simulink library "inp"  (R2021b)
settings: Solver=VariableStepAuto  StartTime=0.0  StopTime=10.0  RelTol=1e-3
undefined symbols (not defined in the file): C_TASK_5MS_S, FALSE, KINP_AcoreReadyToSlp_flg_ovrdflg, KINP_AcoreReadyToSlp_flg_ovrdval, KINP_AllowMovThd_OTA_enum_ovrdflg, KINP_AllowMovThd_OTA_enum_ovrdval, KINP_APSAngleTarget_Deg_ovrdflg, KINP_APSAngleTarget_Deg_ovrdval, KINP_APSDecReq_mps2_ovrdflg, KINP_APSDecReq_mps2_ovrdval, KINP_APSDecReqA_flg_ovrdflg, KINP_APSDecReqA_flg_ovrdval, KINP_APSDFLL_cm_ovrdflg, KINP_APSDFLL_cm_ovrdval, KINP_APSDFLR_cm_ovrdflg, KINP_APSDFLR_cm_ovrdval, KINP_APSDRLL_cm_ovrdflg, KINP_APSDRLL_cm_ovrdval, KINP_APSDRLR_cm_ovrdflg, KINP_APSDRLR_cm_ovrdval, KINP_APSExitCondition_enum_ovrdflg, KINP_APSExitCondition_enum_ovrdval, KINP_APSHWVer_enum_ovrdflg, KINP_APSHWVer_enum_ovrdval, KINP_APSProgressPCT_pct_ovrdflg, KINP_APSProgressPCT_pct_ovrdval, KINP_APSPwrReq_enum_ovrdflg, KINP_APSPwrReq_enum_ovrdval, KINP_APSReq_enum_ovrdflg, KINP_APSReq_enum_ovrdval, KINP_APSRQDisplay_enum_ovrdflg, KINP_APSRQDisplay_enum_ovrdval, KINP_APSRqEPASCtrl_flg_ovrdflg, KINP_APSRqEPASCtrl_flg_ovrdval, KINP_APSShiftPosnReq_enum_ovrdval, KINP_APSShiftPosnReq_enum_ovrflg, KINP_APSSpeedCMD_kph_ovrdval, KINP_APSSpeedCMD_kph_ovrflg, KINP_APSStaSystem_enum_ovrdflg, KINP_APSStaSystem_enum_ovrdval, KINP_APSSWVer_enum_ovrdflg, KINP_APSSWVer_enum_ovrdval, KINP_APSVMCReqA_flg_ovrdval, KINP_APSVMCReqA_flg_ovrflg, KINP_APSVRqEPASCtrl_flg_ovrdflg, KINP_APSVRqEPASCtrl_flg_ovrdval, KINP_AuxBattVolmV_mV_ovrdflg, KINP_AuxBattVolmV_mV_ovrdval, KINP_BTConnectSta_enum_ovrdflg, KINP_BTConnectSta_enum_ovrdval, KINP_CAASSta_enum_ovrdflg, KINP_CAASSta_enum_ovrdval, KINP_CAASVMCReqA_flg_ovrdval, KINP_CAASVMCReqA_flg_ovrflg, KINP_CAN1BusOff_flg_ovrdflg, KINP_CAN1BusOff_flg_ovrdval, KINP_CAN2BusOff_flg_ovrdflg, KINP_CAN2BusOff_flg_ovrdval, KINP_CAN3BusOff_flg_ovrdflg, KINP_CAN3BusOff_flg_ovrdval ... (+158)
libraries: FVT_lib x184, hcu_lib x1
(part 5 of 8)

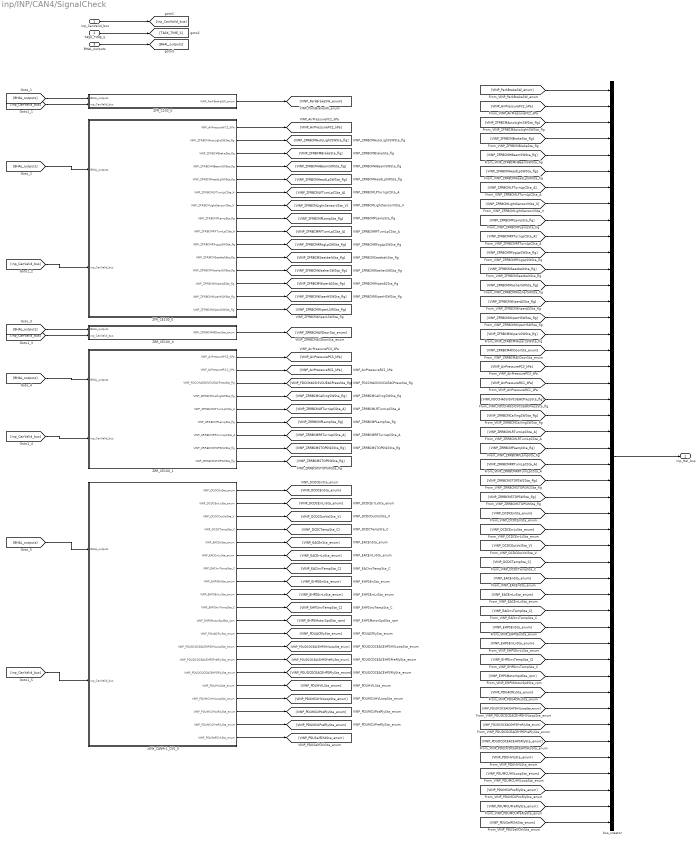
== system inp/INP/CAN4/SignalCheck ==
  inp_CanValid_bus : Inport
  TASK_TIME_S : Inport  Port=2
  BHAL_outputs : Inport  Port=3
  ZFR_C100_0 : Subsystem
  ZFR_CE100_0 : Subsystem
  ZRR_CE100_0 : Subsystem
  ZRR_CE100_1 : Subsystem
  bus_creator : BusCreator  Inputs=46
  zGW_CANRr1_C50_0 : Subsystem
  inp_Hal_bus : Outport
  wires:
  inp_CanValid_bus/1 -> [inp_CanValid_bus]
  TASK_TIME_S/1 -> [TASK_TIME_S]
  BHAL_outputs/1 -> [BHAL_outputs]
  [BHAL_outputs] -> ZFR_C100_0/1(BHAL_outputs)
  [inp_CanValid_bus] -> ZFR_C100_0/2(inp_CanValid_bus)
  ZFR_C100_0/1(VINP_ParkBrakeSW_enum) -> [VINP_ParkBrakeSW_enum]
  [BHAL_outputs] -> ZFR_CE100_0/1(BHAL_outputs)
  [inp_CanValid_bus] -> ZFR_CE100_0/2(inp_CanValid_bus)
  ZFR_CE100_0/1(VINP_AirPressureFC2_kPa) -> [VINP_AirPressureFC2_kPa]
  ZFR_CE100_0/2(VINP_ZFRBCMAutoLightSWSta_flg) -> [VINP_ZFRBCMAutoLightSWSta_flg]
  ZFR_CE100_0/3(VINP_ZFRBCMBrakeSta_flg) -> [VINP_ZFRBCMBrakeSta_flg]
  ZFR_CE100_0/4(VINP_ZFRBCMHBeamSWSta_flg) -> [VINP_ZFRBCMHBeamSWSta_flg]
  ZFR_CE100_0/5(VINP_ZFRBCMHeadLpSWSta_flg) -> [VINP_ZFRBCMHeadLpSWSta_flg]
  ZFR_CE100_0/6(VINP_ZFRBCMLFTurnLpCSta_A) -> [VINP_ZFRBCMLFTurnLpCSta_A]
  ZFR_CE100_0/7(VINP_ZFRBCMLightSensorVSta_V) -> [VINP_ZFRBCMLightSensorVSta_V]
  ZFR_CE100_0/8(VINP_ZFRBCMPLampSta_flg) -> [VINP_ZFRBCMPLampSta_flg]
  ZFR_CE100_0/9(VINP_ZFRBCMRFTurnLpCSta_A) -> [VINP_ZFRBCMRFTurnLpCSta_A]
  ZFR_CE100_0/10(VINP_ZFRBCMRFogLpSWSta_flg) -> [VINP_ZFRBCMRFogLpSWSta_flg]
  ZFR_CE100_0/11(VINP_ZFRBCMSeatbeltSta_flg) -> [VINP_ZFRBCMSeatbeltSta_flg]
  ZFR_CE100_0/12(VINP_ZFRBCMWasherSWSta_flg) -> [VINP_ZFRBCMWasherSWSta_flg]
  ZFR_CE100_0/13(VINP_ZFRBCMWiperASSta_flg) -> [VINP_ZFRBCMWiperASSta_flg]
  ZFR_CE100_0/14(VINP_ZFRBCMWiperHSWSta_flg) -> [VINP_ZFRBCMWiperHSWSta_flg]
  ZFR_CE100_0/15(VINP_ZFRBCMWiperLSWSta_flg) -> [VINP_ZFRBCMWiperLSWSta_flg]
  [BHAL_outputs] -> ZRR_CE100_0/1(BHAL_outputs)
  [inp_CanValid_bus] -> ZRR_CE100_0/2(inp_CanValid_bus)
  ZRR_CE100_0/1(VINP_ZRRBCMAllDoorSta_enum) -> [VINP_ZRRBCMAllDoorSta_enum]
  [BHAL_outputs] -> ZRR_CE100_1/1(BHAL_outputs)
  [inp_CanValid_bus] -> ZRR_CE100_1/2(inp_CanValid_bus)
  ZRR_CE100_1/1(VINP_AirPressurePC3_kPa) -> [VINP_AirPressurePC3_kPa]
  ZRR_CE100_1/2(VINP_AirPressureRC1_kPa) -> [VINP_AirPressureRC1_kPa]
  ZRR_CE100_1/3(VINP_FDCCHASSISVCUEACPressSta_flg) -> [VINP_FDCCHASSISVCUEACPressSta_flg]
  ZRR_CE100_1/4(VINP_ZRRBCMCallingSWSta_flg) -> [VINP_ZRRBCMCallingSWSta_flg]
  ZRR_CE100_1/5(VINP_ZRRBCMLRTurnLpCSta_A) -> [VINP_ZRRBCMLRTurnLpCSta_A]
  ZRR_CE100_1/6(VINP_ZRRBCMPLampSta_flg) -> [VINP_ZRRBCMPLampSta_flg]
  ZRR_CE100_1/7(VINP_ZRRBCMRRTurnLpCSta_A) -> [VINP_ZRRBCMRRTurnLpCSta_A]
  ZRR_CE100_1/8(VINP_ZRRBCMSTOPSW2Sta_flg) -> [VINP_ZRRBCMSTOPSW2Sta_flg]
  ZRR_CE100_1/9(VINP_ZRRBCMSTOPSWSta_flg) -> [VINP_ZRRBCMSTOPSWSta_flg]
  [BHAL_outputs] -> zGW_CANRr1_C50_0/1(BHAL_outputs)
  [inp_CanValid_bus] -> zGW_CANRr1_C50_0/2(inp_CanValid_bus)
  zGW_CANRr1_C50_0/1(VINP_DCDCEnSta_enum) -> [VINP_DCDCEnSta_enum]
  zGW_CANRr1_C50_0/2(VINP_DCDCErrLvSta_enum) -> [VINP_DCDCErrLvSta_enum]
  zGW_CANRr1_C50_0/3(VINP_DCDCOutVolSta_V) -> [VINP_DCDCOutVolSta_V]
  zGW_CANRr1_C50_0/4(VINP_DCDCTempSta_C) -> [VINP_DCDCTempSta_C]
  zGW_CANRr1_C50_0/5(VINP_EACEnSta_enum) -> [VINP_EACEnSta_enum]
  zGW_CANRr1_C50_0/6(VINP_EACErrLvSta_enum) -> [VINP_EACErrLvSta_enum]
  zGW_CANRr1_C50_0/7(VINP_EACInvTempSta_C) -> [VINP_EACInvTempSta_C]
  zGW_CANRr1_C50_0/8(VINP_EHPSEnSta_enum) -> [VINP_EHPSEnSta_enum]
  zGW_CANRr1_C50_0/9(VINP_EHPSErrLvSta_enum) -> [VINP_EHPSErrLvSta_enum]
  zGW_CANRr1_C50_0/10(VINP_EHPSInvTempSta_C) -> [VINP_EHPSInvTempSta_C]
  zGW_CANRr1_C50_0/11(VINP_EHPSMotorSpdSta_rpm) -> [VINP_EHPSMotorSpdSta_rpm]
  zGW_CANRr1_C50_0/12(VINP_PDUACRlySta_enum) -> [VINP_PDUACRlySta_enum]
  zGW_CANRr1_C50_0/13(VINP_PDUDCDCEACEHPSHVLoopSta_enum) -> [VINP_PDUDCDCEACEHPSHVLoopSta_enum]
  zGW_CANRr1_C50_0/14(VINP_PDUDCDCEACEHPSPreRlySta_enum) -> [VINP_PDUDCDCEACEHPSPreRlySta_enum]
  zGW_CANRr1_C50_0/15(VINP_PDUDCDCEACEHPSRlySta_enum) -> [VINP_PDUDCDCEACEHPSRlySta_enum]
  zGW_CANRr1_C50_0/16(VINP_PDUHVILSta_enum) -> [VINP_PDUHVILSta_enum]
  zGW_CANRr1_C50_0/17(VINP_PDUMCUHVLoopSta_enum) -> [VINP_PDUMCUHVLoopSta_enum]
  zGW_CANRr1_C50_0/18(VINP_PDUMCUPosRlySta_enum) -> [VINP_PDUMCUPosRlySta_enum]
  zGW_CANRr1_C50_0/19(VINP_PDUMCUPreRlySta_enum) -> [VINP_PDUMCUPreRlySta_enum]
  zGW_CANRr1_C50_0/20(VINP_PDUSelfChkSta_enum) -> [VINP_PDUSelfChkSta_enum]
  bus_creator/1 -> inp_Hal_bus/1
  [VINP_ParkBrakeSW_enum] -> bus_creator/1
  [VINP_AirPressureFC2_kPa] -> bus_creator/2
  [VINP_ZFRBCMAutoLightSWSta_flg] -> bus_creator/3
  [VINP_ZFRBCMBrakeSta_flg] -> bus_creator/4
  [VINP_ZFRBCMHBeamSWSta_flg] -> bus_creator/5
  [VINP_ZFRBCMHeadLpSWSta_flg] -> bus_creator/6
  [VINP_ZFRBCMLFTurnLpCSta_A] -> bus_creator/7
  [VINP_ZFRBCMLightSensorVSta_V] -> bus_creator/8
  [VINP_ZFRBCMPLampSta_flg] -> bus_creator/9
  [VINP_ZFRBCMRFTurnLpCSta_A] -> bus_creator/10
  [VINP_ZFRBCMRFogLpSWSta_flg] -> bus_creator/11
  [VINP_ZFRBCMSeatbeltSta_flg] -> bus_creator/12
  [VINP_ZFRBCMWasherSWSta_flg] -> bus_creator/13
  [VINP_ZFRBCMWiperASSta_flg] -> bus_creator/14
  [VINP_ZFRBCMWiperHSWSta_flg] -> bus_creator/15
  [VINP_ZFRBCMWiperLSWSta_flg] -> bus_creator/16
  [VINP_ZRRBCMAllDoorSta_enum] -> bus_creator/17
  [VINP_AirPressurePC3_kPa] -> bus_creator/18
  [VINP_AirPressureRC1_kPa] -> bus_creator/19
  [VINP_FDCCHASSISVCUEACPressSta_flg] -> bus_creator/20
  [VINP_ZRRBCMCallingSWSta_flg] -> bus_creator/21
  [VINP_ZRRBCMLRTurnLpCSta_A] -> bus_creator/22
  [VINP_ZRRBCMPLampSta_flg] -> bus_creator/23
  [VINP_ZRRBCMRRTurnLpCSta_A] -> bus_creator/24
  [VINP_ZRRBCMSTOPSW2Sta_flg] -> bus_creator/25
  [VINP_ZRRBCMSTOPSWSta_flg] -> bus_creator/26
  [VINP_DCDCEnSta_enum] -> bus_creator/27
  [VINP_DCDCErrLvSta_enum] -> bus_creator/28
  [VINP_DCDCOutVolSta_V] -> bus_creator/29
  [VINP_DCDCTempSta_C] -> bus_creator/30
  [VINP_EACEnSta_enum] -> bus_creator/31
  [VINP_EACErrLvSta_enum] -> bus_creator/32
  [VINP_EACInvTempSta_C] -> bus_creator/33
  [VINP_EHPSEnSta_enum] -> bus_creator/34
  [VINP_EHPSErrLvSta_enum] -> bus_creator/35
  [VINP_EHPSInvTempSta_C] -> bus_creator/36
  [VINP_EHPSMotorSpdSta_rpm] -> bus_creator/37
  [VINP_PDUACRlySta_enum] -> bus_creator/38
  [VINP_PDUDCDCEACEHPSHVLoopSta_enum] -> bus_creator/39
  [VINP_PDUDCDCEACEHPSPreRlySta_enum] -> bus_creator/40
  [VINP_PDUDCDCEACEHPSRlySta_enum] -> bus_creator/41
  [VINP_PDUHVILSta_enum] -> bus_creator/42
  [VINP_PDUMCUHVLoopSta_enum] -> bus_creator/43
  [VINP_PDUMCUPosRlySta_enum] -> bus_creator/44
  [VINP_PDUMCUPreRlySta_enum] -> bus_creator/45
  [VINP_PDUSelfChkSta_enum] -> bus_creator/46

== system inp/INP/DDM/Subsystem13 ==
  In1 : Inport
  Constant : Constant  Value=KINP_ClearDTCcmd_flg_ovrdval
  Constant1 : Constant  Value=KINP_ClearDTCcmd_flg_ovrdflg
  Switch : Switch  Criteria=u2 ~= 0
  Out1 : Outport
  wires:
  Constant1/1 -> Switch/2
  Constant/1 -> Switch/1
  Switch/1 -> Out1/1
  In1/1 -> Switch/3

== system inp/INP/DKC/Subsystem1 ==
  In1 : Inport
  Constant : Constant  Value=KINP_NFCLidASta_flg_ovrdval
  Constant1 : Constant  Value=KINP_NFCLidASta_flg_ovrdflg
  Switch : Switch  Criteria=u2 ~= 0
  Out1 : Outport
  wires:
  Constant1/1 -> Switch/2
  Constant/1 -> Switch/1
  Switch/1 -> Out1/1
  In1/1 -> Switch/3

== system inp/INP/DKC/Subsystem10 ==
  In1 : Inport
  Constant : Constant  Value=KINP_NFCDoorSta_flg_ovrdval
  Constant1 : Constant  Value=KINP_NFCDoorSta_flg_ovrdflg
  Switch : Switch  Criteria=u2 ~= 0
  Out1 : Outport
  wires:
  Constant1/1 -> Switch/2
  Constant/1 -> Switch/1
  Switch/1 -> Out1/1
  In1/1 -> Switch/3

== system inp/INP/DKC/Subsystem2 ==
  In1 : Inport
  Constant : Constant  Value=KINP_KeyFobAreaU16_enum_ovrdval
  Constant1 : Constant  Value=KINP_KeyFobAreaU16_enum_ovrdflg
  Switch : Switch  Criteria=u2 ~= 0
  Out1 : Outport
  wires:
  Constant1/1 -> Switch/2
  Constant/1 -> Switch/1
  Switch/1 -> Out1/1
  In1/1 -> Switch/3

== system inp/INP/DKC/Subsystem3 ==
  In1 : Inport
  Constant : Constant  Value=KINP_UIDButtonCmd_enum_ovrdval
  Constant1 : Constant  Value=KINP_UIDButtonCmd_enum_ovrdflg
  Switch : Switch  Criteria=u2 ~= 0
  Out1 : Outport
  wires:
  Constant1/1 -> Switch/2
  Constant/1 -> Switch/1
  Switch/1 -> Out1/1
  In1/1 -> Switch/3

== system inp/INP/DKC/Subsystem4 ==
  In1 : Inport
  Constant : Constant  Value=KINP_BTConnectSta_enum_ovrdval
  Constant1 : Constant  Value=KINP_BTConnectSta_enum_ovrdflg
  Switch : Switch  Criteria=u2 ~= 0
  Out1 : Outport
  wires:
  Constant1/1 -> Switch/2
  Constant/1 -> Switch/1
  Switch/1 -> Out1/1
  In1/1 -> Switch/3

== system inp/INP/DKC/Subsystem5 ==
  In1 : Inport
  Constant : Constant  Value=KINP_UIDBatVoltx1000_V_ovrdval
  Constant1 : Constant  Value=KINP_UIDBatVoltx1000_V_ovrdflg
  Switch : Switch  Criteria=u2 ~= 0
  Out1 : Outport
  wires:
  Switch/1 -> Out1/1
  Constant/1 -> Switch/1
  Constant1/1 -> Switch/2
  In1/1 -> Switch/3

== system inp/INP/DKC/Subsystem6 ==
  In1 : Inport
  Constant : Constant  Value=KINP_DKCBTRSSI_dB_ovrdval
  Constant1 : Constant  Value=KINP_DKCBTRSSI_dB_ovrdflg
  Switch : Switch  Criteria=u2 ~= 0
  Out1 : Outport
  wires:
  Constant1/1 -> Switch/2
  Constant/1 -> Switch/1
  Switch/1 -> Out1/1
  In1/1 -> Switch/3

== system inp/INP/GPIO/Analog ==
  BHAL_outputs : Inport
  TASK_TIME_S : Inport  Port=2
  AccelPedal1Vol_V : FVT_lib/inp/ad_signal_template  SystemSampleTime=-1  VariantActivationTime=update diagram  Latency=0  AutoFrameSizeCalculation=off
      link override defval: Value=KINP_AccelPedal1Vol_V_defval
      link override fftdec: Value=KINP_AccelPedal1Vol_V_fftdec
      link override fftinc: Value=KINP_AccelPedal1Vol_V_fftinc
      link override fftlim: Value=KINP_AccelPedal1Vol_V_fftlim
      link override limlow: Value=KINP_AccelPedal1Vol_V_limlow
      link override limupr: Value=KINP_AccelPedal1Vol_V_limupr
      link override ovrdflg: Value=KINP_AccelPedal1Vol_V_ovrdflg
      link override ovrdval: Value=KINP_AccelPedal1Vol_V_ovrdval
      link override srvcflg: Value=KINP_AccelPedal1Vol_V_srvcflg
      link override srvcval: Value=KINP_AccelPedal1Vol_V_srvcval
      link override tcfilt: Value=KINP_AccelPedal1Vol_V_tcfilt
  AccelPedal2Vol_V : FVT_lib/inp/ad_signal_template  SystemSampleTime=-1  VariantActivationTime=update diagram  Latency=0  AutoFrameSizeCalculation=off
      link override defval: Value=KINP_AccelPedal2Vol_V_defval
      link override fftdec: Value=KINP_AccelPedal2Vol_V_fftdec
      link override fftinc: Value=KINP_AccelPedal2Vol_V_fftinc
      link override fftlim: Value=KINP_AccelPedal2Vol_V_fftlim
      link override limlow: Value=KINP_AccelPedal2Vol_V_limlow
      link override limupr: Value=KINP_AccelPedal2Vol_V_limupr
      link override ovrdflg: Value=KINP_AccelPedal2Vol_V_ovrdflg
      link override ovrdval: Value=KINP_AccelPedal2Vol_V_ovrdval
      link override srvcflg: Value=KINP_AccelPedal2Vol_V_srvcflg
      link override srvcval: Value=KINP_AccelPedal2Vol_V_srvcval
      link override tcfilt: Value=KINP_AccelPedal2Vol_V_tcfilt
  Bus Selector : BusSelector  OutputSignals=VHAL_AccelPedal1Vol_V
  Bus Selector1 : BusSelector  OutputSignals=VHAL_AccelPedal2Vol_V
  Constant{,1..3} (4 alike) : Constant  Value=FALSE
  VINP_AccelPedal1VolShortHigh_enum : Outport
  VINP_AccelPedal1VolShortLow_enum : Outport  Port=2
  VINP_AccelPedal1Vol_V : Outport  Port=3
  VINP_AccelPedal1VolValid_flg : Outport  Port=4
  VINP_AccelPedal2VolShortHigh_enum : Outport  Port=5
  VINP_AccelPedal2VolShortLow_enum : Outport  Port=6
  VINP_AccelPedal2Vol_V : Outport  Port=7
  VINP_AccelPedal2VolValid_flg : Outport  Port=8
  wires:
  BHAL_outputs/1 -> [BHAL_outputs]
  TASK_TIME_S/1 -> [TASK_TIME_S]
  AccelPedal1Vol_V/1 -> VINP_AccelPedal1VolShortHigh_enum/1  "VINP_AccelPedal1VolShortHigh_enum"
  AccelPedal1Vol_V/2 -> VINP_AccelPedal1VolShortLow_enum/1  "VINP_AccelPedal1VolShortLow_enum"
  AccelPedal1Vol_V/3 -> VINP_AccelPedal1Vol_V/1  "VINP_AccelPedal1Vol_V"
  AccelPedal1Vol_V/4 -> VINP_AccelPedal1VolValid_flg/1  "VINP_AccelPedal1VolValid_flg"
  AccelPedal2Vol_V/1 -> VINP_AccelPedal2VolShortHigh_enum/1  "VINP_AccelPedal2VolShortHigh_enum"
  AccelPedal2Vol_V/2 -> VINP_AccelPedal2VolShortLow_enum/1  "VINP_AccelPedal2VolShortLow_enum"
  AccelPedal2Vol_V/3 -> VINP_AccelPedal2Vol_V/1  "VINP_AccelPedal2Vol_V"
  AccelPedal2Vol_V/4 -> VINP_AccelPedal2VolValid_flg/1  "VINP_AccelPedal2VolValid_flg"
  [TASK_TIME_S] -> AccelPedal1Vol_V/4
  Constant1/1 -> AccelPedal1Vol_V/3
  Constant/1 -> AccelPedal1Vol_V/2
  [BHAL_outputs] -> Bus Selector/1
  Bus Selector/1 -> AccelPedal1Vol_V/1  "<VHAL_AccelPedal1Vol_V>"
  Bus Selector1/1 -> AccelPedal2Vol_V/1  "<VHAL_AccelPedal2Vol_V>"
  [BHAL_outputs] -> Bus Selector1/1
  Constant2/1 -> AccelPedal2Vol_V/2
  Constant3/1 -> AccelPedal2Vol_V/3
  [TASK_TIME_S] -> AccelPedal2Vol_V/4

== system inp/INP/GPIO/Digital ==
  BHAL_outputs : Inport
  AlcoholPass : FVT_lib/inp/di_signal_template  SystemSampleTime=-1  VariantActivationTime=update diagram  Latency=0  AutoFrameSizeCalculation=off
      link override debdec: Value=KINP_AlcoholPass_flg_debdec
      link override debinc: Value=KINP_AlcoholPass_flg_debinc
      link override deblim: Value=KINP_AlcoholPass_flg_deblim
      link override inverse: Value=KINP_AlcoholPass_flg_inverse
      link override ovrdflg: Value=KINP_AlcoholPass_flg_ovrdflg
      link override ovrdval: Value=KINP_AlcoholPass_flg_ovrdval
      link override srvcflg: Value=KINP_AlcoholPass_flg_srvcflg
      link override srvcval: Value=KINP_AlcoholPass_flg_srvcval
  BmsAplus : FVT_lib/inp/di_signal_template  SystemSampleTime=-1  VariantActivationTime=update diagram  Latency=0  AutoFrameSizeCalculation=off
      link override debdec: Value=KINP_BmsAplus_flg_debdec
      link override debinc: Value=KINP_BmsAplus_flg_debinc
      link override deblim: Value=KINP_BmsAplus_flg_deblim
      link override inverse: Value=KINP_BmsAplus_flg_inverse
      link override ovrdflg: Value=KINP_BmsAplus_flg_ovrdflg
      link override ovrdval: Value=KINP_BmsAplus_flg_ovrdval
      link override srvcflg: Value=KINP_BmsAplus_flg_srvcflg
      link override srvcval: Value=KINP_BmsAplus_flg_srvcval
  BrakeLampSW : FVT_lib/inp/di_signal_template  SystemSampleTime=-1  VariantActivationTime=update diagram  Latency=0  AutoFrameSizeCalculation=off
      link override debdec: Value=KINP_BrakeLampSW_flg_debdec
      link override debinc: Value=KINP_BrakeLampSW_flg_debinc
      link override deblim: Value=KINP_BrakeLampSW_flg_deblim
      link override inverse: Value=KINP_BrakeLampSW_flg_inverse
      link override ovrdflg: Value=KINP_BrakeLampSW_flg_ovrdflg
      link override ovrdval: Value=KINP_BrakeLampSW_flg_ovrdval
      link override srvcflg: Value=KINP_BrakeLampSW_flg_srvcflg
      link override srvcval: Value=KINP_BrakeLampSW_flg_srvcval
  BrakeSWGPIO : FVT_lib/inp/di_signal_template  SystemSampleTime=-1  VariantActivationTime=update diagram  Latency=0  AutoFrameSizeCalculation=off
      link override debdec: Value=KINP_BrakeSWGPIO_flg_debdec
      link override debinc: Value=KINP_BrakeSWGPIO_flg_debinc
      link override deblim: Value=KINP_BrakeSWGPIO_flg_deblim
      link override inverse: Value=KINP_BrakeSWGPIO_flg_inverse
      link override ovrdflg: Value=KINP_BrakeSWGPIO_flg_ovrdflg
      link override ovrdval: Value=KINP_BrakeSWGPIO_flg_ovrdval
      link override srvcflg: Value=KINP_BrakeSWGPIO_flg_srvcflg
      link override srvcval: Value=KINP_BrakeSWGPIO_flg_srvcval
  CrashSignalGPIO : FVT_lib/inp/di_signal_template  SystemSampleTime=-1  VariantActivationTime=update diagram  Latency=0  AutoFrameSizeCalculation=off
      link override debdec: Value=KINP_CrashSignalGPIO_flg_debdec
      link override debinc: Value=KINP_CrashSignalGPIO_flg_debinc
      link override deblim: Value=KINP_CrashSignalGPIO_flg_deblim
      link override inverse: Value=KINP_CrashSignalGPIO_flg_inverse
      link override ovrdflg: Value=KINP_CrashSignalGPIO_flg_ovrdflg
      link override ovrdval: Value=KINP_CrashSignalGPIO_flg_ovrdval
      link override srvcflg: Value=KINP_CrashSignalGPIO_flg_srvcflg
      link override srvcval: Value=KINP_CrashSignalGPIO_flg_srvcval
  EmergencyExitSW : FVT_lib/inp/di_signal_template  SystemSampleTime=-1  VariantActivationTime=update diagram  Latency=0  AutoFrameSizeCalculation=off
      link override debdec: Value=KINP_EmergencyExitSW_flg_debdec
      link override debinc: Value=KINP_EmergencyExitSW_flg_debinc
      link override deblim: Value=KINP_EmergencyExitSW_flg_deblim
      link override inverse: Value=KINP_EmergencyExitSW_flg_inverse
      link override ovrdflg: Value=KINP_EmergencyExitSW_flg_ovrdflg
      link override ovrdval: Value=KINP_EmergencyExitSW_flg_ovrdval
      link override srvcflg: Value=KINP_EmergencyExitSW_flg_srvcflg
      link override srvcval: Value=KINP_EmergencyExitSW_flg_srvcval
  FrontDoorSW : FVT_lib/inp/di_signal_template  SystemSampleTime=-1  VariantActivationTime=update diagram  Latency=0  AutoFrameSizeCalculation=off
      link override debdec: Value=KINP_FrontDoorSW_flg_debdec
      link override debinc: Value=KINP_FrontDoorSW_flg_debinc
      link override deblim: Value=KINP_FrontDoorSW_flg_deblim
      link override inverse: Value=KINP_FrontDoorSW_flg_inverse
      link override ovrdflg: Value=KINP_FrontDoorSW_flg_ovrdflg
      link override ovrdval: Value=KINP_FrontDoorSW_flg_ovrdval
      link override srvcflg: Value=KINP_FrontDoorSW_flg_srvcflg
      link override srvcval: Value=KINP_FrontDoorSW_flg_srvcval
  HazardSW : FVT_lib/inp/di_signal_template  SystemSampleTime=-1  VariantActivationTime=update diagram  Latency=0  AutoFrameSizeCalculation=off
      link override debdec: Value=KINP_HazardSW_flg_debdec
      link override debinc: Value=KINP_HazardSW_flg_debinc
      link override deblim: Value=KINP_HazardSW_flg_deblim
      link override inverse: Value=KINP_HazardSW_flg_inverse
      link override ovrdflg: Value=KINP_HazardSW_flg_ovrdflg
      link override ovrdval: Value=KINP_HazardSW_flg_ovrdval
      link override srvcflg: Value=KINP_HazardSW_flg_srvcflg
      link override srvcval: Value=KINP_HazardSW_flg_srvcval
  LeftTurnSW : FVT_lib/inp/di_signal_template  SystemSampleTime=-1  VariantActivationTime=update diagram  Latency=0  AutoFrameSizeCalculation=off
      link override debdec: Value=KINP_LeftTurnSW_flg_debdec
      link override debinc: Value=KINP_LeftTurnSW_flg_debinc
      link override deblim: Value=KINP_LeftTurnSW_flg_deblim
      link override inverse: Value=KINP_LeftTurnSW_flg_inverse
      link override ovrdflg: Value=KINP_LeftTurnSW_flg_ovrdflg
      link override ovrdval: Value=KINP_LeftTurnSW_flg_ovrdval
      link override srvcflg: Value=KINP_LeftTurnSW_flg_srvcflg
      link override srvcval: Value=KINP_LeftTurnSW_flg_srvcval
  MidDoorSW : FVT_lib/inp/di_signal_template  SystemSampleTime=-1  VariantActivationTime=update diagram  Latency=0  AutoFrameSizeCalculation=off
      link override debdec: Value=KINP_MidDoorSW_flg_debdec
      link override debinc: Value=KINP_MidDoorSW_flg_debinc
      link override deblim: Value=KINP_MidDoorSW_flg_deblim
      link override inverse: Value=KINP_MidDoorSW_flg_inverse
      link override ovrdflg: Value=KINP_MidDoorSW_flg_ovrdflg
      link override ovrdval: Value=KINP_MidDoorSW_flg_ovrdval
      link override srvcflg: Value=KINP_MidDoorSW_flg_srvcflg
      link override srvcval: Value=KINP_MidDoorSW_flg_srvcval
  OSDoorSwClose : FVT_lib/inp/di_signal_template  SystemSampleTime=-1  VariantActivationTime=update diagram  Latency=0  AutoFrameSizeCalculation=off
      link override debdec: Value=KINP_OSDoorSwClose_flg_debdec
      link override debinc: Value=KINP_OSDoorSwClose_flg_debinc
      link override deblim: Value=KINP_OSDoorSwClose_flg_deblim
      link override inverse: Value=KINP_OSDoorSwClose_flg_inverse
      link override ovrdflg: Value=KINP_OSDoorSwClose_flg_ovrdflg
      link override ovrdval: Value=KINP_OSDoorSwClose_flg_ovrdval
      link override srvcflg: Value=KINP_OSDoorSwClose_flg_srvcflg
      link override srvcval: Value=KINP_OSDoorSwClose_flg_srvcval
  OSDoorSwOpen : FVT_lib/inp/di_signal_template  SystemSampleTime=-1  VariantActivationTime=update diagram  Latency=0  AutoFrameSizeCalculation=off
      link override debdec: Value=KINP_OSDoorSwOpen_flg_debdec
      link override debinc: Value=KINP_OSDoorSwOpen_flg_debinc
      link override deblim: Value=KINP_OSDoorSwOpen_flg_deblim
      link override inverse: Value=KINP_OSDoorSwOpen_flg_inverse
      link override ovrdflg: Value=KINP_OSDoorSwOpen_flg_ovrdflg
      link override ovrdval: Value=KINP_OSDoorSwOpen_flg_ovrdval
      link override srvcflg: Value=KINP_OSDoorSwOpen_flg_srvcflg
      link override srvcval: Value=KINP_OSDoorSwOpen_flg_srvcval
  PushButton : FVT_lib/inp/di_signal_template  SystemSampleTime=-1  VariantActivationTime=update diagram  Latency=0  AutoFrameSizeCalculation=off
      link override debdec: Value=KINP_PushButton_flg_debdec
      link override debinc: Value=KINP_PushButton_flg_debinc
      link override deblim: Value=KINP_PushButton_flg_deblim
      link override inverse: Value=KINP_PushButton_flg_inverse
      link override ovrdflg: Value=KINP_PushButton_flg_ovrdflg
      link override ovrdval: Value=KINP_PushButton_flg_ovrdval
      link override srvcflg: Value=KINP_PushButton_flg_srvcflg
      link override srvcval: Value=KINP_PushButton_flg_srvcval
  RightTurnSW : FVT_lib/inp/di_signal_template  SystemSampleTime=-1  VariantActivationTime=update diagram  Latency=0  AutoFrameSizeCalculation=off
      link override debdec: Value=KINP_RightTurnSW_flg_debdec
      link override debinc: Value=KINP_RightTurnSW_flg_debinc
      link override deblim: Value=KINP_RightTurnSW_flg_deblim
      link override inverse: Value=KINP_RightTurnSW_flg_inverse
      link override ovrdflg: Value=KINP_RightTurnSW_flg_ovrdflg
      link override ovrdval: Value=KINP_RightTurnSW_flg_ovrdval
      link override srvcflg: Value=KINP_RightTurnSW_flg_srvcflg
      link override srvcval: Value=KINP_RightTurnSW_flg_srvcval
  SeatSW : FVT_lib/inp/di_signal_template  SystemSampleTime=-1  VariantActivationTime=update diagram  Latency=0  AutoFrameSizeCalculation=off
      link override debdec: Value=KINP_SeatSW_flg_debdec
      link override debinc: Value=KINP_SeatSW_flg_debinc
      link override deblim: Value=KINP_SeatSW_flg_deblim
      link override inverse: Value=KINP_SeatSW_flg_inverse
      link override ovrdflg: Value=KINP_SeatSW_flg_ovrdflg
      link override ovrdval: Value=KINP_SeatSW_flg_ovrdval
      link override srvcflg: Value=KINP_SeatSW_flg_srvcflg
      link override srvcval: Value=KINP_SeatSW_flg_srvcval
  TailgateSW : FVT_lib/inp/di_signal_template  SystemSampleTime=-1  VariantActivationTime=update diagram  Latency=0  AutoFrameSizeCalculation=off
      link override debdec: Value=KINP_TailgateSW_flg_debdec
      link override debinc: Value=KINP_TailgateSW_flg_debinc
      link override deblim: Value=KINP_TailgateSW_flg_deblim
      link override inverse: Value=KINP_TailgateSW_flg_inverse
      link override ovrdflg: Value=KINP_TailgateSW_flg_ovrdflg
      link override ovrdval: Value=KINP_TailgateSW_flg_ovrdval
      link override srvcflg: Value=KINP_TailgateSW_flg_srvcflg
      link override srvcval: Value=KINP_TailgateSW_flg_srvcval
  TrunkHanSW : FVT_lib/inp/di_signal_template  SystemSampleTime=-1  VariantActivationTime=update diagram  Latency=0  AutoFrameSizeCalculation=off
      link override debdec: Value=KINP_TrunkHanSW_flg_debdec
      link override debinc: Value=KINP_TrunkHanSW_flg_debinc
      link override deblim: Value=KINP_TrunkHanSW_flg_deblim
      link override inverse: Value=KINP_TrunkHanSW_flg_inverse
      link override ovrdflg: Value=KINP_TrunkHanSW_flg_ovrdflg
      link override ovrdval: Value=KINP_TrunkHanSW_flg_ovrdval
      link override srvcflg: Value=KINP_TrunkHanSW_flg_srvcflg
      link override srvcval: Value=KINP_TrunkHanSW_flg_srvcval
  slr_VINP_BrakeLampSW_flg : BusSelector  OutputSignals=VHAL_BrakeLampSW_flg
  slr_VINP_BrakeSWGPIO_flg : BusSelector  OutputSignals=VHAL_BrakeSWGPIO_flg
  slr_VINP_CentralDoorLockSW_flg : BusSelector  OutputSignals=VHAL_OSDoorSwOpen_flg
  slr_VINP_CentralDoorLockSW_flg1 : BusSelector  OutputSignals=VHAL_OSDoorSwClose_flg
  slr_VINP_CrashSignalGPIO_flg : BusSelector  OutputSignals=VHAL_CrashSignalGPIO_flg
  slr_VINP_CrashSignalGPIO_flg1 : BusSelector  OutputSignals=VHAL_PushButton_flg
  slr_VINP_CrashSignalGPIO_flg2 : BusSelector  OutputSignals=VHAL_AlcoholPass_flg
  slr_VINP_CrashSignalGPIO_flg3 : BusSelector  OutputSignals=VHAL_BmsAplus_flg
  slr_VINP_DrDoorSW_flg : BusSelector  OutputSignals=VHAL_LeftTurnSW_flg
  slr_VINP_HazardSW_flg : BusSelector  OutputSignals=VHAL_HazardSW_flg
  slr_VINP_HoodSW_flg : BusSelector  OutputSignals=VHAL_EmergencyExitSW_flg
  slr_VINP_PsDoorSW_flg : BusSelector  OutputSignals=VHAL_RightTurnSW_flg
  slr_VINP_RLDoorSW_flg : BusSelector  OutputSignals=VHAL_MidDoorSW_flg
  slr_VINP_RRDoorSW_flg : BusSelector  OutputSignals=VHAL_FrontDoorSW_flg
  slr_VINP_SeatSW_flg : BusSelector  OutputSignals=VHAL_SeatSW_flg
  slr_VINP_TailgateSW_flg : BusSelector  OutputSignals=VHAL_TailgateSW_flg
  slr_VINP_TrunkHanSW_flg : BusSelector  OutputSignals=VHAL_TrunkHanSW_flg
  VINP_BrakeSWGPIO_flg : Outport
  VINP_EmergencyExitSW_flg : Outport  Port=2
  VINP_TailgateSW_flg : Outport  Port=3
  VINP_LeftTurnSW_flg : Outport  Port=4
  VINP_RightTurnSW_flg : Outport  Port=5
  VINP_FrontDoorSW_flg : Outport  Port=6
  VINP_MidDoorSW_flg : Outport  Port=7
  VINP_OSDoorSwOpen_flg : Outport  Port=8
  VINP_OSDoorSwClose_flg : Outport  Port=9
  VINP_HazardSW_flg : Outport  Port=10
  VINP_BrakeLampSW_flg : Outport  Port=11
  VINP_TrunkHanSW_flg : Outport  Port=12
  VINP_SeatSW_flg : Outport  Port=13
  VINP_CrashSignalGPIO_flg : Outport  Port=14
  VINP_PushButton_flg : Outport  Port=15
  VINP_AlcoholPass_flg : Outport  Port=16
  VINP_BmsAplus_flg : Outport  Port=17
  wires:
  BHAL_outputs/1 -> [BHAL_outputs]
  BrakeSWGPIO/1 -> VINP_BrakeSWGPIO_flg/1  "VINP_BrakeSWGPIO_flg"
  [BHAL_outputs] -> slr_VINP_BrakeSWGPIO_flg/1
  slr_VINP_BrakeSWGPIO_flg/1 -> BrakeSWGPIO/1  "<VHAL_BrakeSWGPIO_flg>"
  EmergencyExitSW/1 -> VINP_EmergencyExitSW_flg/1  "VINP_EmergencyExitSW_flg"
  [BHAL_outputs] -> slr_VINP_HoodSW_flg/1
  slr_VINP_HoodSW_flg/1 -> EmergencyExitSW/1  "<VHAL_EmergencyExitSW_flg>"
  TailgateSW/1 -> VINP_TailgateSW_flg/1  "VINP_TailgateSW_flg"
  [BHAL_outputs] -> slr_VINP_TailgateSW_flg/1
  slr_VINP_TailgateSW_flg/1 -> TailgateSW/1  "<VHAL_TailgateSW_flg>"
  LeftTurnSW/1 -> VINP_LeftTurnSW_flg/1  "VINP_LeftTurnSW_flg"
  [BHAL_outputs] -> slr_VINP_DrDoorSW_flg/1
  slr_VINP_DrDoorSW_flg/1 -> LeftTurnSW/1  "<VHAL_LeftTurnSW_flg>"
  RightTurnSW/1 -> VINP_RightTurnSW_flg/1  "VINP_RightTurnSW_flg"
  [BHAL_outputs] -> slr_VINP_PsDoorSW_flg/1
  slr_VINP_PsDoorSW_flg/1 -> RightTurnSW/1  "<VHAL_RightTurnSW_flg>"
  FrontDoorSW/1 -> VINP_FrontDoorSW_flg/1  "VINP_FrontDoorSW_flg"
  [BHAL_outputs] -> slr_VINP_RRDoorSW_flg/1
  slr_VINP_RRDoorSW_flg/1 -> FrontDoorSW/1  "<VHAL_FrontDoorSW_flg>"
  MidDoorSW/1 -> VINP_MidDoorSW_flg/1  "VINP_MidDoorSW_flg"
  [BHAL_outputs] -> slr_VINP_RLDoorSW_flg/1
  slr_VINP_RLDoorSW_flg/1 -> MidDoorSW/1  "<VHAL_MidDoorSW_flg>"
  OSDoorSwOpen/1 -> VINP_OSDoorSwOpen_flg/1  "VINP_OSDoorSwOpen_flg"
  [BHAL_outputs] -> slr_VINP_CentralDoorLockSW_flg/1
  slr_VINP_CentralDoorLockSW_flg/1 -> OSDoorSwOpen/1  "<VHAL_OSDoorSwOpen_flg>"
  HazardSW/1 -> VINP_HazardSW_flg/1  "VINP_HazardSW_flg"
  [BHAL_outputs] -> slr_VINP_HazardSW_flg/1
  slr_VINP_HazardSW_flg/1 -> HazardSW/1  "<VHAL_HazardSW_flg>"
  BrakeLampSW/1 -> VINP_BrakeLampSW_flg/1  "VINP_BrakeLampSW_flg"
  [BHAL_outputs] -> slr_VINP_BrakeLampSW_flg/1
  slr_VINP_BrakeLampSW_flg/1 -> BrakeLampSW/1  "<VHAL_BrakeLampSW_flg>"
  TrunkHanSW/1 -> VINP_TrunkHanSW_flg/1  "VINP_TrunkHanSW_flg"
  [BHAL_outputs] -> slr_VINP_TrunkHanSW_flg/1
  slr_VINP_TrunkHanSW_flg/1 -> TrunkHanSW/1  "<VHAL_TrunkHanSW_flg>"
  SeatSW/1 -> VINP_SeatSW_flg/1  "VINP_SeatSW_flg"
  [BHAL_outputs] -> slr_VINP_SeatSW_flg/1
  slr_VINP_SeatSW_flg/1 -> SeatSW/1  "<VHAL_SeatSW_flg>"
  [BHAL_outputs] -> slr_VINP_CrashSignalGPIO_flg/1
  slr_VINP_CrashSignalGPIO_flg/1 -> CrashSignalGPIO/1  "<VHAL_CrashSignalGPIO_flg>"
  CrashSignalGPIO/1 -> VINP_CrashSignalGPIO_flg/1  "VINP_CrashSignalGPIO_flg"
  [BHAL_outputs] -> slr_VINP_CentralDoorLockSW_flg1/1
  slr_VINP_CentralDoorLockSW_flg1/1 -> OSDoorSwClose/1  "<VHAL_OSDoorSwClose_flg>"
  OSDoorSwClose/1 -> VINP_OSDoorSwClose_flg/1  "VINP_OSDoorSwClose_flg"
  PushButton/1 -> VINP_PushButton_flg/1  "VINP_PushButton_flg"
  AlcoholPass/1 -> VINP_AlcoholPass_flg/1  "VINP_AlcoholPass_flg"
  BmsAplus/1 -> VINP_BmsAplus_flg/1  "VINP_BmsAplus_flg"
  [BHAL_outputs] -> slr_VINP_CrashSignalGPIO_flg1/1
  [BHAL_outputs] -> slr_VINP_CrashSignalGPIO_flg2/1
  [BHAL_outputs] -> slr_VINP_CrashSignalGPIO_flg3/1
  slr_VINP_CrashSignalGPIO_flg1/1 -> PushButton/1  "<VHAL_PushButton_flg>"
  slr_VINP_CrashSignalGPIO_flg2/1 -> AlcoholPass/1  "<VHAL_AlcoholPass_flg>"
  slr_VINP_CrashSignalGPIO_flg3/1 -> BmsAplus/1  "<VHAL_BmsAplus_flg>"

== system inp/INP/IMU/Subsystem1 ==
  In1 : Inport
  Constant : Constant  Value=KINP_MemOffsetGyroY_raw16_ovrdval
  Constant1 : Constant  Value=KINP_MemOffsetGyroY_raw16_ovrdflg
  Switch : Switch  Criteria=u2 ~= 0
  Out1 : Outport
  wires:
  Switch/1 -> Out1/1
  Constant/1 -> Switch/1
  Constant1/1 -> Switch/2
  In1/1 -> Switch/3

== system inp/INP/IMU/Subsystem10 ==
  In1 : Inport
  Constant : Constant  Value=KINP_SensingAccZ_raw16_ovrdval
  Constant1 : Constant  Value=KINP_SensingAccZ_raw16_ovrdflg
  Switch : Switch  Criteria=u2 ~= 0
  Out1 : Outport
  wires:
  Constant1/1 -> Switch/2
  Constant/1 -> Switch/1
  Switch/1 -> Out1/1
  In1/1 -> Switch/3

== system inp/INP/IMU/Subsystem11 ==
  In1 : Inport
  Constant : Constant  Value=KINP_SensingAccY_raw16_ovrdval
  Constant1 : Constant  Value=KINP_SensingAccY_raw16_ovrdflg
  Switch : Switch  Criteria=u2 ~= 0
  Out1 : Outport
  wires:
  Switch/1 -> Out1/1
  Constant/1 -> Switch/1
  Constant1/1 -> Switch/2
  In1/1 -> Switch/3

== system inp/INP/IMU/Subsystem15 ==
  In1 : Inport
  Constant : Constant  Value=KINP_MemOffsetGyroX_raw16_ovrdval
  Constant1 : Constant  Value=KINP_MemOffsetGyroX_raw16_ovrdflg
  Switch : Switch  Criteria=u2 ~= 0
  Out1 : Outport
  wires:
  Constant1/1 -> Switch/2
  Constant/1 -> Switch/1
  Switch/1 -> Out1/1
  In1/1 -> Switch/3

== system inp/INP/IMU/Subsystem2 ==
  In1 : Inport
  Constant : Constant  Value=KINP_MemOffsetAccX_raw16_ovrdval
  Constant1 : Constant  Value=KINP_MemOffsetAccX_raw16_ovrdflg
  Switch : Switch  Criteria=u2 ~= 0
  Out1 : Outport
  wires:
  Constant1/1 -> Switch/2
  Constant/1 -> Switch/1
  Switch/1 -> Out1/1
  In1/1 -> Switch/3

== system inp/INP/IMU/Subsystem3 ==
  In1 : Inport
  Constant : Constant  Value=KINP_MemOffsetGyroZ_raw16_ovrdval
  Constant1 : Constant  Value=KINP_MemOffsetGyroZ_raw16_ovrdflg
  Switch : Switch  Criteria=u2 ~= 0
  Out1 : Outport
  wires:
  Switch/1 -> Out1/1
  Constant/1 -> Switch/1
  Constant1/1 -> Switch/2
  In1/1 -> Switch/3

== system inp/INP/IMU/Subsystem4 ==
  In1 : Inport
  Constant : Constant  Value=KINP_MemOffsetAccZ_raw16_ovrdval
  Constant1 : Constant  Value=KINP_MemOffsetAccZ_raw16_ovrdflg
  Switch : Switch  Criteria=u2 ~= 0
  Out1 : Outport
  wires:
  Switch/1 -> Out1/1
  Constant/1 -> Switch/1
  Constant1/1 -> Switch/2
  In1/1 -> Switch/3

== system inp/INP/IMU/Subsystem5 ==
  In1 : Inport
  Constant : Constant  Value=KINP_MemOffsetAccY_raw16_ovrdval
  Constant1 : Constant  Value=KINP_MemOffsetAccY_raw16_ovrdflg
  Switch : Switch  Criteria=u2 ~= 0
  Out1 : Outport
  wires:
  Constant1/1 -> Switch/2
  Constant/1 -> Switch/1
  Switch/1 -> Out1/1
  In1/1 -> Switch/3

== system inp/INP/IMU/Subsystem6 ==
  In1 : Inport
  Constant : Constant  Value=KINP_SensingGyroY_raw16_ovrdval
  Constant1 : Constant  Value=KINP_SensingGyroY_raw16_ovrdflg
  Switch : Switch  Criteria=u2 ~= 0
  Out1 : Outport
  wires:
  Constant1/1 -> Switch/2
  Constant/1 -> Switch/1
  Switch/1 -> Out1/1
  In1/1 -> Switch/3

== system inp/INP/IMU/Subsystem7 ==
  In1 : Inport
  Constant : Constant  Value=KINP_SensingGyroX_raw16_ovrdval
  Constant1 : Constant  Value=KINP_SensingGyroX_raw16_ovrdflg
  Switch : Switch  Criteria=u2 ~= 0
  Out1 : Outport
  wires:
  Switch/1 -> Out1/1
  Constant/1 -> Switch/1
  Constant1/1 -> Switch/2
  In1/1 -> Switch/3

== system inp/INP/IMU/Subsystem8 ==
  In1 : Inport
  Constant : Constant  Value=KINP_SensingAccX_raw16_ovrdval
  Constant1 : Constant  Value=KINP_SensingAccX_raw16_ovrdflg
  Switch : Switch  Criteria=u2 ~= 0
  Out1 : Outport
  wires:
  Switch/1 -> Out1/1
  Constant/1 -> Switch/1
  Constant1/1 -> Switch/2
  In1/1 -> Switch/3

== system inp/INP/IMU/Subsystem9 ==
  In1 : Inport
  Constant : Constant  Value=KINP_SensingGyroZ_raw16_ovrdval
  Constant1 : Constant  Value=KINP_SensingGyroZ_raw16_ovrdflg
  Switch : Switch  Criteria=u2 ~= 0
  Out1 : Outport
  wires:
  Constant1/1 -> Switch/2
  Constant/1 -> Switch/1
  Switch/1 -> Out1/1
  In1/1 -> Switch/3

== system inp/INP/SYS/Subsystem ==
  In1 : Inport
  Constant : Constant  Value=KINP_AuxBattVolmV_mV_ovrdflg
  Constant1 : Constant  Value=KINP_AuxBattVolmV_mV_ovrdval
  Switch : Switch  Criteria=u2 > Threshold
  Out1 : Outport
  wires:
  Constant1/1 -> Switch/1
  Constant/1 -> Switch/2
  In1/1 -> Switch/3
  Switch/1 -> Out1/1

== system inp/INP/SYS/Subsystem1 ==
  In1 : Inport
  Constant : Constant  Value=KINP_NetworkReqCalled_flg_ovrdflg
  Constant1 : Constant  Value=KINP_NetworkReqCalled_flg_ovrdval
  Switch : Switch  Criteria=u2 > Threshold
  Out1 : Outport
  wires:
  Constant1/1 -> Switch/1
  Constant/1 -> Switch/2
  In1/1 -> Switch/3
  Switch/1 -> Out1/1

== system inp/INP/SYS/Subsystem10 ==
  In1 : Inport
  Constant : Constant  Value=KINP_CAN3BusOff_flg_ovrdflg
  Constant1 : Constant  Value=KINP_CAN3BusOff_flg_ovrdval
  Switch : Switch  Criteria=u2 > Threshold
  Out1 : Outport
  wires:
  Constant1/1 -> Switch/1
  Constant/1 -> Switch/2
  In1/1 -> Switch/3
  Switch/1 -> Out1/1

== system inp/INP/SYS/Subsystem11 ==
  In1 : Inport
  Constant : Constant  Value=KINP_CAN6BusOff_flg_ovrdflg
  Constant1 : Constant  Value=KINP_CAN6BusOff_flg_ovrdval
  Switch : Switch  Criteria=u2 > Threshold
  Out1 : Outport
  wires:
  Switch/1 -> Out1/1
  In1/1 -> Switch/3
  Constant/1 -> Switch/2
  Constant1/1 -> Switch/1

== system inp/INP/SYS/Subsystem12 ==
  In1 : Inport
  Constant : Constant  Value=KINP_CAN4BusOff_flg_ovrdflg
  Constant1 : Constant  Value=KINP_CAN4BusOff_flg_ovrdval
  Switch : Switch  Criteria=u2 > Threshold
  Out1 : Outport
  wires:
  Switch/1 -> Out1/1
  In1/1 -> Switch/3
  Constant/1 -> Switch/2
  Constant1/1 -> Switch/1

== system inp/INP/SYS/Subsystem13 ==
  In1 : Inport
  Constant : Constant  Value=KINP_CAN5BusOff_flg_ovrdflg
  Constant1 : Constant  Value=KINP_CAN5BusOff_flg_ovrdval
  Switch : Switch  Criteria=u2 > Threshold
  Out1 : Outport
  wires:
  Constant1/1 -> Switch/1
  Constant/1 -> Switch/2
  In1/1 -> Switch/3
  Switch/1 -> Out1/1

== system inp/INP/SYS/Subsystem2 ==
  In1 : Inport
  Constant : Constant  Value=KINP_Pedal1Ref5V_V_ovrdflg
  Constant1 : Constant  Value=KINP_Pedal1Ref5V_V_ovrdval
  Switch : Switch  Criteria=u2 > Threshold
  Out1 : Outport
  wires:
  Switch/1 -> Out1/1
  In1/1 -> Switch/3
  Constant/1 -> Switch/2
  Constant1/1 -> Switch/1

== system inp/INP/SYS/Subsystem3 ==
  In1 : Inport
  Constant : Constant  Value=KINP_Pedal2Ref5V_V_ovrdflg
  Constant1 : Constant  Value=KINP_Pedal2Ref5V_V_ovrdval
  Switch : Switch  Criteria=u2 > Threshold
  Out1 : Outport
  wires:
  Constant1/1 -> Switch/1
  Constant/1 -> Switch/2
  In1/1 -> Switch/3
  Switch/1 -> Out1/1

== system inp/INP/SYS/Subsystem4 ==
  In1 : Inport
  Constant : Constant  Value=KINP_PwrReq_OTA_enum_ovrdval
  Constant1 : Constant  Value=KINP_PwrReq_OTA_enum_ovrdflg
  Switch : Switch  Criteria=u2 ~= 0
  Out1 : Outport
  wires:
  Constant1/1 -> Switch/2
  Constant/1 -> Switch/1
  In1/1 -> Switch/3
  Switch/1 -> Out1/1

== system inp/INP/SYS/Subsystem5 ==
  In1 : Inport
  Constant : Constant  Value=KINP_AllowMovThd_OTA_enum_ovrdval
  Constant1 : Constant  Value=KINP_AllowMovThd_OTA_enum_ovrdflg
  Switch : Switch  Criteria=u2 ~= 0
  Out1 : Outport
  wires:
  Switch/1 -> Out1/1
  In1/1 -> Switch/3
  Constant/1 -> Switch/1
  Constant1/1 -> Switch/2

== system inp/INP/SYS/Subsystem6 ==
  In1 : Inport
  Constant : Constant  Value=KINP_EvccAplusPwrUpReq_flg_ovrdval
  Constant1 : Constant  Value=KINP_EvccAplusPwrUpReq_flg_ovrdflg
  Switch : Switch  Criteria=u2 ~= 0
  Out1 : Outport
  wires:
  Constant1/1 -> Switch/2
  Constant/1 -> Switch/1
  In1/1 -> Switch/3
  Switch/1 -> Out1/1

== system inp/INP/SYS/Subsystem7 ==
  In1 : Inport
  Constant : Constant  Value=KINP_AcoreReadyToSlp_flg_ovrdval
  Constant1 : Constant  Value=KINP_AcoreReadyToSlp_flg_ovrdflg
  Switch : Switch  Criteria=u2 ~= 0
  Out1 : Outport
  wires:
  Switch/1 -> Out1/1
  In1/1 -> Switch/3
  Constant/1 -> Switch/1
  Constant1/1 -> Switch/2

== system inp/INP/SYS/Subsystem8 ==
  In1 : Inport
  Constant : Constant  Value=KINP_CAN1BusOff_flg_ovrdflg
  Constant1 : Constant  Value=KINP_CAN1BusOff_flg_ovrdval
  Switch : Switch  Criteria=u2 > Threshold
  Out1 : Outport
  wires:
  Constant1/1 -> Switch/1
  Constant/1 -> Switch/2
  In1/1 -> Switch/3
  Switch/1 -> Out1/1

== system inp/INP/SYS/Subsystem9 ==
  In1 : Inport
  Constant : Constant  Value=KINP_CAN2BusOff_flg_ovrdflg
  Constant1 : Constant  Value=KINP_CAN2BusOff_flg_ovrdval
  Switch : Switch  Criteria=u2 > Threshold
  Out1 : Outport
  wires:
  Switch/1 -> Out1/1
  In1/1 -> Switch/3
  Constant/1 -> Switch/2
  Constant1/1 -> Switch/1

== system inp/INP/TPMS/Subsystem ==
  In1 : Inport
  Constant : Constant  Value=KINP_TPMSDataIn_flg_ovrdval
  Constant1 : Constant  Value=KINP_TPMSDataIn_flg_ovrdflg
  Switch : Switch  Criteria=u2 ~= 0
  Out1 : Outport
  wires:
  Switch/1 -> Out1/1
  In1/1 -> Switch/3
  Constant/1 -> Switch/1
  Constant1/1 -> Switch/2

== system inp/INP/TPMS/Subsystem1 ==
  In1 : Inport
  Constant : Constant  Value=KINP_TPMSID_raw_ovrdflg
  Constant1 : Constant  Value=KINP_TPMSID_raw_ovrdval
  Switch : Switch  Criteria=u2 ~= 0
  Out1 : Outport
  wires:
  Constant/1 -> Switch/2
  Constant1/1 -> Switch/1
  Switch/1 -> Out1/1
  In1/1 -> Switch/3

== system inp/INP/TPMS/Subsystem10 ==
  In1 : Inport
  Constant : Constant  Value=KINP_TPMSStorge_flg_ovrflg
  Constant1 : Constant  Value=KINP_TPMSStorge_flg_ovrdval
  Switch : Switch  Criteria=u2 ~= 0
  Out1 : Outport
  wires:
  Constant1/1 -> Switch/1
  Constant/1 -> Switch/2
  In1/1 -> Switch/3
  Switch/1 -> Out1/1

== system inp/INP/TPMS/Subsystem11 ==
  In1 : Inport
  Constant : Constant  Value=KINP_LFID_raw_ovrflg
  Constant1 : Constant  Value=KINP_LFID_raw_ovrdval
  Switch : Switch  Criteria=u2 ~= 0
  Out1 : Outport
  wires:
  Switch/1 -> Out1/1
  In1/1 -> Switch/3
  Constant/1 -> Switch/2
  Constant1/1 -> Switch/1

== system inp/INP/TPMS/Subsystem12 ==
  In1 : Inport
  Constant : Constant  Value=KINP_RFID_raw_ovrdval
  Constant1 : Constant  Value=KINP_RFID_raw_ovrdval
  Switch : Switch  Criteria=u2 ~= 0
  Out1 : Outport
  wires:
  Constant1/1 -> Switch/1
  Constant/1 -> Switch/2
  In1/1 -> Switch/3
  Switch/1 -> Out1/1

== system inp/INP/TPMS/Subsystem13 ==
  In1 : Inport
  Constant : Constant  Value=KINP_LRID_raw_ovrdval
  Constant1 : Constant  Value=KINP_LRID_raw_ovrdval
  Switch : Switch  Criteria=u2 ~= 0
  Out1 : Outport
  wires:
  Switch/1 -> Out1/1
  In1/1 -> Switch/3
  Constant/1 -> Switch/2
  Constant1/1 -> Switch/1

== system inp/INP/TPMS/Subsystem14 ==
  In1 : Inport
  Constant : Constant  Value=KINP_RRID_raw_ovrdval
  Constant1 : Constant  Value=KINP_RRID_raw_ovrdval
  Switch : Switch  Criteria=u2 ~= 0
  Out1 : Outport
  wires:
  Constant1/1 -> Switch/1
  Constant/1 -> Switch/2
  In1/1 -> Switch/3
  Switch/1 -> Out1/1

== system inp/INP/TPMS/Subsystem2 ==
  In1 : Inport
  Constant : Constant  Value=KINP_TPMSPressure_raw_ovrdflg
  Constant1 : Constant  Value=KINP_TPMSPressure_raw_ovrdval
  Switch : Switch  Criteria=u2 ~= 0
  Out1 : Outport
  wires:
  Constant/1 -> Switch/2
  Constant1/1 -> Switch/1
  Switch/1 -> Out1/1
  In1/1 -> Switch/3

== system inp/INP/TPMS/Subsystem3 ==
  In1 : Inport
  Constant : Constant  Value=KINP_TPMSTemp_raw_ovrdflg
  Constant1 : Constant  Value=KINP_TPMSTemp_raw_ovrdval
  Switch : Switch  Criteria=u2 ~= 0
  Out1 : Outport
  wires:
  Constant/1 -> Switch/2
  Constant1/1 -> Switch/1
  Switch/1 -> Out1/1
  In1/1 -> Switch/3

== system inp/INP/TPMS/Subsystem4 ==
  In1 : Inport
  Constant : Constant  Value=KINP_TPMSSta_enum_ovrdflg
  Constant1 : Constant  Value=KINP_TPMSSta_enum_ovrdval
  Switch : Switch  Criteria=u2 ~= 0
  Out1 : Outport
  wires:
  Constant/1 -> Switch/2
  Constant1/1 -> Switch/1
  Switch/1 -> Out1/1
  In1/1 -> Switch/3

== system inp/INP/TPMS/Subsystem5 ==
  In1 : Inport
  Constant : Constant  Value=KINP_TPMSPressureMi_raw_ovrdflg
  Constant1 : Constant  Value=KINP_TPMSPressureMi_raw_ovrdval
  Switch : Switch  Criteria=u2 ~= 0
  Out1 : Outport
  wires:
  Constant/1 -> Switch/2
  Constant1/1 -> Switch/1
  Switch/1 -> Out1/1
  In1/1 -> Switch/3

== system inp/INP/TPMS/Subsystem6 ==
  In1 : Inport
  Constant : Constant  Value=KINP_TPMSCRC_crc_ovrdflg
  Constant1 : Constant  Value=KINP_TPMSCRC_crc_ovrdval
  Switch : Switch  Criteria=u2 ~= 0
  Out1 : Outport
  wires:
  Constant/1 -> Switch/2
  Constant1/1 -> Switch/1
  Switch/1 -> Out1/1
  In1/1 -> Switch/3

== system inp/INP/TPMS/Subsystem7 ==
  In1 : Inport
  Constant : Constant  Value=KINP_TPMSCRCCalc_crc_ovrdflg
  Constant1 : Constant  Value=KINP_TPMSCRCCalc_crc_ovrdval
  Switch : Switch  Criteria=u2 ~= 0
  Out1 : Outport
  wires:
  Constant/1 -> Switch/2
  Constant1/1 -> Switch/1
  Switch/1 -> Out1/1
  In1/1 -> Switch/3

== system inp/INP/TPMS/Subsystem8 ==
  In1 : Inport
  Constant : Constant  Value=KINP_TPMSFAT_flg_ovrflg
  Constant1 : Constant  Value=KINP_TPMSFAT_flg_ovrdval
  Switch : Switch  Criteria=u2 ~= 0
  Out1 : Outport
  wires:
  Switch/1 -> Out1/1
  In1/1 -> Switch/3
  Constant1/1 -> Switch/1
  Constant/1 -> Switch/2

== system inp/INP/TPMS/Subsystem9 ==
  In1 : Inport
  Constant : Constant  Value=KINP_TPMSBattLow_flg_ovrflg
  Constant1 : Constant  Value=KINP_TPMSBattLow_flg_ovrdval
  Switch : Switch  Criteria=u2 ~= 0
  Out1 : Outport
  wires:
  Switch/1 -> Out1/1
  In1/1 -> Switch/3
  Constant/1 -> Switch/2
  Constant1/1 -> Switch/1

== system inp/INP/CAN1/SignalCheck/AC_BTMS_C1000_0 ==
  BHAL_outputs : Inport
  inp_CanValid_bus : Inport  Port=2
  ACAmbTemp : FVT_lib/inp/can_signal_template  SystemSampleTime=-1  VariantActivationTime=update diagram  Latency=0  AutoFrameSizeCalculation=off
      link override defval: Value=KINP_ACAmbTemp_C_defval
      link override ovrdflg: Value=KINP_ACAmbTemp_C_ovrdflg
      link override ovrdval: Value=KINP_ACAmbTemp_C_ovrdval
  Terminator_1 : Terminator
  True_VHAL_ACAmbTemp_C : Constant  Value=TRUE  OutDataTypeStr=boolean
  slr1_1 : BusSelector  OutputSignals=VINP_CANMsgValidACBTMSC10000_flg
  slr_VHAL_ACAmbTemp_C : BusSelector  OutputSignals=VHAL_ACAmbTemp_C
  VINP_ACAmbTemp_C : Outport
  wires:
  BHAL_outputs/1 -> [BHAL_outputs]
  inp_CanValid_bus/1 -> [inp_CanValid_bus]
  [BHAL_outputs] -> slr_VHAL_ACAmbTemp_C/1
  slr_VHAL_ACAmbTemp_C/1 -> ACAmbTemp/1  "<VHAL_ACAmbTemp_C>"
  True_VHAL_ACAmbTemp_C/1 -> ACAmbTemp/2
  [inp_CanValid_bus] -> slr1_1/1
  slr1_1/1 -> ACAmbTemp/3  "<VINP_CANMsgValidACBTMSC10000_flg>"
  ACAmbTemp/1 -> VINP_ACAmbTemp_C/1  "VINP_ACAmbTemp_C"
  ACAmbTemp/2 -> Terminator_1/1

== system inp/INP/CAN1/SignalCheck/AC_BTMS_C1000_1 ==
  BHAL_outputs : Inport
  inp_CanValid_bus : Inport  Port=2
  ACFanSpdSta : FVT_lib/inp/can_signal_template  SystemSampleTime=-1  VariantActivationTime=update diagram  Latency=0  AutoFrameSizeCalculation=off
      link override defval: Value=KINP_ACFanSpdSta_enum_defval
      link override ovrdflg: Value=KINP_ACFanSpdSta_enum_ovrdflg
      link override ovrdval: Value=KINP_ACFanSpdSta_enum_ovrdval
  Terminator_1 : Terminator
  True_VHAL_ACFanSpdSta_enum : Constant  Value=TRUE  OutDataTypeStr=boolean
  slr1_1 : BusSelector  OutputSignals=VINP_CANMsgValidACBTMSC10001_flg
  slr_VHAL_ACFanSpdSta_enum : BusSelector  OutputSignals=VHAL_ACFanSpdSta_enum
  VINP_ACFanSpdSta_enum : Outport
  wires:
  BHAL_outputs/1 -> [BHAL_outputs]
  inp_CanValid_bus/1 -> [inp_CanValid_bus]
  [BHAL_outputs] -> slr_VHAL_ACFanSpdSta_enum/1
  slr_VHAL_ACFanSpdSta_enum/1 -> ACFanSpdSta/1  "<VHAL_ACFanSpdSta_enum>"
  True_VHAL_ACFanSpdSta_enum/1 -> ACFanSpdSta/2
  [inp_CanValid_bus] -> slr1_1/1
  slr1_1/1 -> ACFanSpdSta/3  "<VINP_CANMsgValidACBTMSC10001_flg>"
  ACFanSpdSta/1 -> VINP_ACFanSpdSta_enum/1  "VINP_ACFanSpdSta_enum"
  ACFanSpdSta/2 -> Terminator_1/1

== system inp/INP/CAN1/SignalCheck/AC_BTMS_C1000_4 ==
  BHAL_outputs : Inport
  inp_CanValid_bus : Inport  Port=2
  TM2BFaultCode : FVT_lib/inp/can_signal_template  SystemSampleTime=-1  VariantActivationTime=update diagram  Latency=0  AutoFrameSizeCalculation=off
      link override defval: Value=KINP_TM2BFaultCode_enum_defval
      link override ovrdflg: Value=KINP_TM2BFaultCode_enum_ovrdflg
      link override ovrdval: Value=KINP_TM2BFaultCode_enum_ovrdval
  Terminator_1 : Terminator
  True_VHAL_TM2BFaultCode_enum : Constant  Value=TRUE  OutDataTypeStr=boolean
  slr1_1 : BusSelector  OutputSignals=VINP_CANMsgValidACBTMSC10004_flg
  slr_VHAL_TM2BFaultCode_enum : BusSelector  OutputSignals=VHAL_TM2BFaultCode_enum
  VINP_TM2BFaultCode_enum : Outport
  wires:
  BHAL_outputs/1 -> [BHAL_outputs]
  inp_CanValid_bus/1 -> [inp_CanValid_bus]
  [BHAL_outputs] -> slr_VHAL_TM2BFaultCode_enum/1
  slr_VHAL_TM2BFaultCode_enum/1 -> TM2BFaultCode/1  "<VHAL_TM2BFaultCode_enum>"
  True_VHAL_TM2BFaultCode_enum/1 -> TM2BFaultCode/2
  [inp_CanValid_bus] -> slr1_1/1
  slr1_1/1 -> TM2BFaultCode/3  "<VINP_CANMsgValidACBTMSC10004_flg>"
  TM2BFaultCode/1 -> VINP_TM2BFaultCode_enum/1  "VINP_TM2BFaultCode_enum"
  TM2BFaultCode/2 -> Terminator_1/1

== system inp/INP/CAN1/SignalCheck/AC_BTMS_C5000_0 ==
  BHAL_outputs : Inport
  inp_CanValid_bus : Inport  Port=2
  ACTempSetSta : FVT_lib/inp/can_signal_template  SystemSampleTime=-1  VariantActivationTime=update diagram  Latency=0  AutoFrameSizeCalculation=off
      link override defval: Value=KINP_ACTempSetSta_C_defval
      link override ovrdflg: Value=KINP_ACTempSetSta_C_ovrdflg
      link override ovrdval: Value=KINP_ACTempSetSta_C_ovrdval
  Terminator_1 : Terminator
  True_VHAL_ACTempSetSta_C : Constant  Value=TRUE  OutDataTypeStr=boolean
  slr1_1 : BusSelector  OutputSignals=VINP_CANMsgValidACBTMSC50000_flg
  slr_VHAL_ACTempSetSta_C : BusSelector  OutputSignals=VHAL_ACTempSetSta_C
  VINP_ACTempSetSta_C : Outport
  wires:
  BHAL_outputs/1 -> [BHAL_outputs]
  inp_CanValid_bus/1 -> [inp_CanValid_bus]
  [BHAL_outputs] -> slr_VHAL_ACTempSetSta_C/1
  slr_VHAL_ACTempSetSta_C/1 -> ACTempSetSta/1  "<VHAL_ACTempSetSta_C>"
  True_VHAL_ACTempSetSta_C/1 -> ACTempSetSta/2
  [inp_CanValid_bus] -> slr1_1/1
  slr1_1/1 -> ACTempSetSta/3  "<VINP_CANMsgValidACBTMSC50000_flg>"
  ACTempSetSta/1 -> VINP_ACTempSetSta_C/1  "VINP_ACTempSetSta_C"
  ACTempSetSta/2 -> Terminator_1/1
